simulink model "sampleModel1553"  (R2023a)
settings: Solver=VariableStepAuto  StartTime=0.0  StopTime=10.0  RelTol=1e-3
libraries: hdlsllib x5, simulink x2
settings Model: Creator=user1  LastModifiedBy=user1

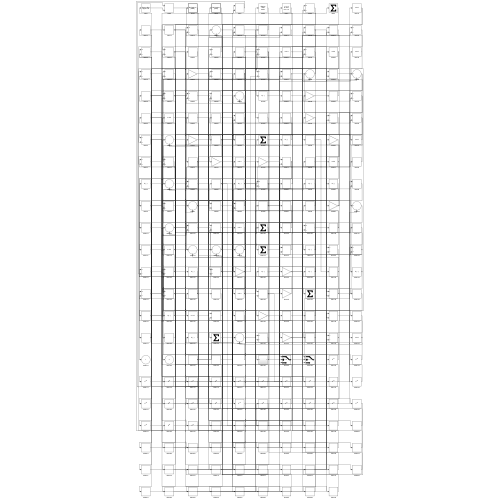
[thumbnail: Simulink's stored preview of the top-level diagram]
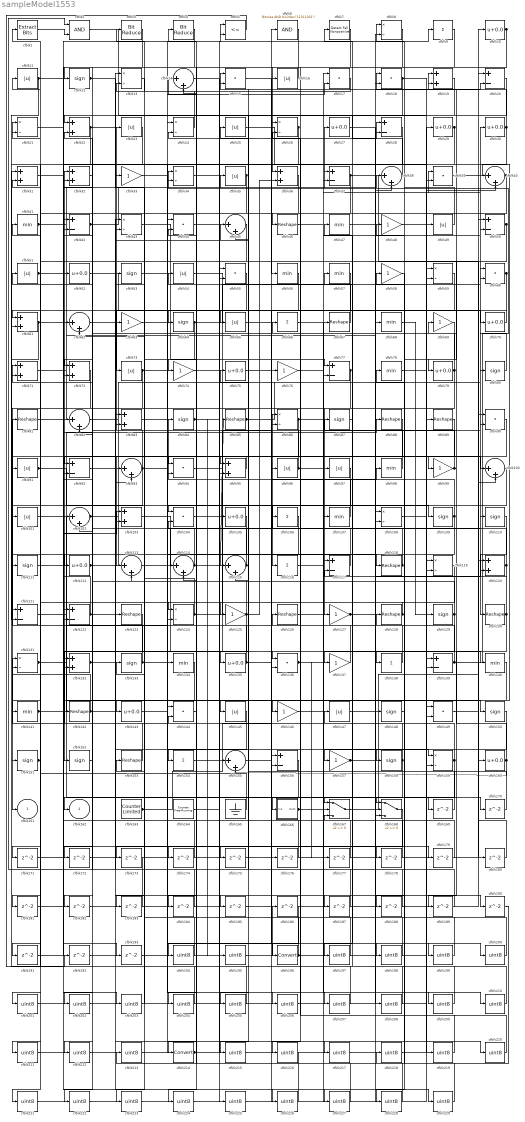
== system sampleModel1553 ==
  cfblk1 : simulink/Logic and Bit Operations/Extract Bits  bitsToExtract=Upper half  numBits=8  bitIdxRange=[0 7]  outScalingMode=Preserve fixed-point scaling
      settings: LibrarySourceBlock=|
      | hdlsllib/Logic and Bit
      | Operations/Extract Bits
  cfblk{10,27,29..30,52,70,75,79,105,112,135,143,160} (13 alike) : Bias  Bias=0.0  SaturateOnIntegerOverflow=off
  cfblk{14,38,40,45,62,82,93,100,102,113..115,155} (13 alike) : Sum  Inputs=|++
  cfblk{11,16,23,25,35,49,51,54,65,73,91,96..97,101,145,147} (16 alike) : Abs  SaturateOnIntegerOverflow=off
  cfblk{19,22,31..32,36,61,71..72,83,95,103,120,132} (13 alike) : Sum
  cfblk{15,17..18,39,44,55,60,90,94,104,136,144,149} (13 alike) : DotProduct  OutDataTypeStr=Inherit: Inherit via internal rule
  cfblk{9,66,106,116,138,154} (6 alike) : Sum  Inputs=+
  cfblk{41,47,56..57,68,78,98,107,134,140..141} (11 alike) : MinMax
  cfblk{8,13,21,24,26,34,43,59,86,108,119,124,131,159} (14 alike) : Product  Inputs=*/  RndMeth=Zero  SaturateOnIntegerOverflow=on
  cfblk{12,53,64,80,84,87,109..111,129,133,148,150..152,158} (16 alike) : Signum
  cfblk{20,28,37,42,50,77,92,117,121..122,139,156} (12 alike) : Sum  Inputs=+-
  cfblk{46,67,81,85,88..89,118,123,126,128,130,142,153} (13 alike) : Reshape
  cfblk{33,48,58,63,69,74,76,99,125,127,137,146,157} (13 alike) : Gain
  cfblk163 : hdlsllib/Sources/Counter Limited  uplimit=7  tsamp=-1
  cfblk164 : hdlsllib/Sources/Counter Free-Running  NumBits=16  tsamp=-1
  cfblk165 : Ground
  cfblk166 : Subsystem
      settings: LibrarySourceBlock=|
      | hdlsllib/Ports &
      | Subsystems/Subsystem
  cfblk167 : Switch  SaturateOnIntegerOverflow=off  InputSameDT=off
  cfblk168 : Switch  SaturateOnIntegerOverflow=off  InputSameDT=off
  cfblk{169..193} (25 alike) : Delay  SampleTime=1
  cfblk{194..195,197..213,215..229} (34 alike) : DataTypeConversion  OutDataTypeStr=uint8  SaturateOnIntegerOverflow=off  RndMeth=Floor
  cfblk196 : DataTypeConversion  SaturateOnIntegerOverflow=off  RndMeth=Floor
  cfblk2 : Logic  AllPortsSameDT=off  OutDataTypeStr=boolean
  cfblk214 : DataTypeConversion  SaturateOnIntegerOverflow=off  RndMeth=Floor
  cfblk3 : hdlsllib/Logic and Bit Operations/Bit Reduce  mode=AND
  cfblk4 : hdlsllib/Logic and Bit Operations/Bit Reduce  mode=AND
  cfblk5 : RelationalOperator  Operator=<=  OutDataTypeStr=boolean  InputSameDT=off
  cfblk6 : simulink/Logic and Bit Operations/Bitwise Operator  logicop=AND  UseBitMask=on  BitMask=bin2dec('11011001')  BitMaskRealWorld=Stored Integer
      settings: LibrarySourceBlock=|
      | hdlsllib/Logic and Bit
      | Operations/Bitwise
      | Operator
  cfblk7 : hdlsllib/Logic and Bit Operations/Detect Fall Nonpositive  vinit=0  OutDataTypeStr=boolean
  cfblk161 : Outport  VectorParamsAs1DForOutWhenUnconnected=off
  cfblk162 : Outport  Port=2  VectorParamsAs1DForOutWhenUnconnected=off
  wires:
  cfblk70/1 -> cfblk61/1
  cfblk84/1 -> cfblk187/1, cfblk195/1
  cfblk77/1 -> cfblk127/1, cfblk124/2
  cfblk139/1 -> cfblk34/1, cfblk103/2
  cfblk73/1 -> cfblk161/1, cfblk199/1
  cfblk54/1 -> cfblk138/1
  cfblk39/1 -> cfblk145/1
  cfblk12/1 -> cfblk217/1, cfblk226/1
  cfblk68/1 -> cfblk129/1
  cfblk26/1 -> cfblk191/1, cfblk205/1, cfblk211/1
  cfblk16/1 -> cfblk12/1
  cfblk122/1 -> cfblk32/1, cfblk123/1
  cfblk98/1 -> cfblk23/1
  cfblk130/1 -> cfblk30/1, cfblk189/1
  cfblk111/1 -> cfblk146/1
  cfblk2/1 -> cfblk119/1
  cfblk22/1 -> cfblk150/1, cfblk93/2, cfblk121/2
  cfblk72/1 -> cfblk151/1
  cfblk103/1 -> cfblk136/1
  cfblk43/1 -> cfblk77/1
  cfblk114/1 -> cfblk85/1, cfblk53/1
  cfblk96/1 -> cfblk75/1, cfblk50/2, cfblk60/2
  cfblk6/1 -> cfblk36/1
  cfblk74/1 -> cfblk9/1
  cfblk158/1 -> cfblk131/1, cfblk184/1
  cfblk143/1 -> cfblk110/1
  cfblk50/1 -> cfblk79/1, cfblk221/1
  cfblk131/1 -> cfblk88/1, cfblk103/1
  cfblk51/1 -> cfblk139/2, cfblk193/1
  cfblk81/1 -> cfblk27/1
  cfblk29/1 -> cfblk46/1, cfblk34/2
  cfblk107/1 -> cfblk84/1
  cfblk15/1 -> cfblk56/1
  cfblk57/1 -> cfblk64/1
  cfblk101/1 -> cfblk167/1
  cfblk75/1 -> cfblk100/1
  cfblk27/1 -> cfblk68/1
  cfblk167/1 -> cfblk50/1
  cfblk7/1 -> cfblk166/1(In1)
  cfblk41/1 -> cfblk13/1, cfblk5/2, cfblk227/1
  cfblk100/1 -> cfblk116/1
  cfblk119/1 -> cfblk141/1
  cfblk69/1 -> cfblk158/1
  cfblk55/1 -> cfblk73/1
  cfblk159/1 -> cfblk62/1, cfblk188/1
  cfblk37/1 -> cfblk160/1, cfblk72/1
  cfblk121/1 -> cfblk143/1
  cfblk123/1 -> cfblk152/1
  cfblk137/1 -> cfblk66/1
  cfblk124/1 -> cfblk6/1, cfblk62/2, cfblk37/1
  cfblk133/1 -> cfblk81/1, cfblk17/2
  cfblk23/1 -> cfblk92/1
  cfblk49/1 -> cfblk18/1
  cfblk19/1 -> cfblk107/1
  cfblk89/1 -> cfblk91/1
  cfblk83/1 -> cfblk38/1
  cfblk164/1 -> cfblk115/1
  cfblk1/1 -> cfblk2/2
  cfblk144/1 -> cfblk4/1
  cfblk56/1 -> cfblk162/1
  cfblk150/1 -> cfblk157/1
  cfblk78/1 -> cfblk140/1
  cfblk128/1 -> cfblk125/1, cfblk78/1
  cfblk97/1 -> cfblk104/1
  cfblk141/1 -> cfblk24/1, cfblk35/1
  cfblk46/1 -> cfblk28/1
  cfblk99/1 -> cfblk69/1, cfblk45/2
  cfblk85/1 -> cfblk49/1, cfblk200/1
  cfblk165/1 -> cfblk41/1
  cfblk35/1 -> cfblk154/1, cfblk224/1
  cfblk38/1 -> cfblk7/1
  cfblk60/1 -> cfblk112/1, cfblk86/2
  cfblk18/1 -> cfblk89/1, cfblk215/1
  cfblk135/1 -> cfblk98/1, cfblk21/1
  cfblk11/1 -> cfblk61/2, cfblk39/2
  cfblk138/1 -> cfblk128/1
  cfblk8/1 -> cfblk124/1
  cfblk166/1(Out1) -> cfblk90/2, cfblk26/2
  cfblk120/1 -> cfblk86/1, cfblk117/2
  cfblk118/1 -> cfblk51/1, cfblk87/1
  cfblk61/1 -> cfblk111/1, cfblk99/1, cfblk71/2, cfblk179/1
  cfblk17/1 -> cfblk13/2
  cfblk33/1 -> cfblk196/1
  cfblk82/1 -> cfblk10/1
  cfblk67/1 -> cfblk54/1
  cfblk148/1 -> cfblk8/1
  cfblk25/1 -> cfblk38/2
  cfblk153/1 -> cfblk11/1
  cfblk112/1 -> cfblk67/1, cfblk92/2
  cfblk109/1 -> cfblk115/2, cfblk48/1, cfblk15/2
  cfblk151/1 -> cfblk131/2, cfblk121/1
  cfblk132/1 -> cfblk159/1, cfblk168/3
  cfblk142/1 -> cfblk168/1, cfblk21/2
  cfblk152/1 -> cfblk82/1
  cfblk110/1 -> cfblk130/1
  cfblk116/1 -> cfblk80/1
  cfblk9/1 -> cfblk94/1
  cfblk126/1 -> cfblk149/2
  cfblk93/1 -> cfblk101/1, cfblk5/1, cfblk71/1
  cfblk129/1 -> cfblk137/1, cfblk113/2
  cfblk40/1 -> cfblk135/1, cfblk65/1
  cfblk113/1 -> cfblk100/2
  cfblk80/1 -> cfblk60/1
  cfblk64/1 -> cfblk37/2, cfblk207/1, cfblk223/1
  cfblk160/1 -> cfblk19/1, cfblk155/2
  cfblk20/1 -> cfblk102/2
  cfblk136/1 -> cfblk40/1, cfblk177/1
  cfblk86/1 -> cfblk170/1, cfblk171/1
  cfblk3/1 -> cfblk22/1
  cfblk42/1 -> cfblk16/1, cfblk70/1
  cfblk48/1 -> cfblk40/2
  cfblk53/1 -> cfblk118/1
  cfblk115/1 -> cfblk32/2, cfblk25/1
  cfblk28/1 -> cfblk94/2
  cfblk163/1 -> cfblk96/1, cfblk28/2
  cfblk45/1 -> cfblk74/1
  cfblk94/1 -> cfblk148/1
  cfblk79/1 -> cfblk42/1, cfblk132/2
  cfblk30/1 -> cfblk132/1, cfblk15/1
  cfblk106/1 -> cfblk214/1
  cfblk147/1 -> cfblk39/1
  cfblk157/1 -> cfblk20/2, cfblk19/2
  cfblk88/1 -> cfblk113/1
  cfblk10/1 -> cfblk142/1, cfblk114/2
  cfblk87/1 -> cfblk57/1
  cfblk52/1 -> cfblk139/1
  cfblk102/1 -> cfblk43/1, cfblk109/1
  cfblk24/1 -> cfblk3/1
  cfblk95/1 -> cfblk93/1
  cfblk71/1 -> cfblk8/2
  cfblk91/1 -> cfblk155/1, cfblk95/1
  cfblk127/1 -> cfblk120/2, cfblk169/1
  cfblk117/1 -> cfblk83/2
  cfblk155/1 -> cfblk136/2
  cfblk4/1 -> cfblk122/2
  cfblk125/1 -> cfblk52/1, cfblk36/2, cfblk182/1
  cfblk169/1 -> cfblk43/2
  cfblk170/1 -> cfblk24/2
  cfblk171/1 -> cfblk77/2
  cfblk32/1 -> cfblk172/1
  cfblk172/1 -> cfblk90/1
  cfblk168/1 -> cfblk173/1
  cfblk173/1 -> cfblk2/1
  cfblk21/1 -> cfblk174/1
  cfblk174/1 -> cfblk122/1
  cfblk92/1 -> cfblk175/1
  cfblk175/1 -> cfblk18/2
  cfblk65/1 -> cfblk176/1
  cfblk176/1 -> cfblk102/1
  cfblk177/1 -> cfblk22/2
  cfblk146/1 -> cfblk178/1
  cfblk178/1 -> cfblk167/2
  cfblk179/1 -> cfblk167/3
  cfblk149/1 -> cfblk180/1
  cfblk180/1 -> cfblk20/1
  cfblk36/1 -> cfblk181/1
  cfblk181/1 -> cfblk114/1
  cfblk182/1 -> cfblk95/2
  cfblk13/1 -> cfblk183/1
  cfblk183/1 -> cfblk83/1
  cfblk184/1 -> cfblk82/2
  cfblk62/1 -> cfblk185/1
  cfblk185/1 -> cfblk120/1
  cfblk187/1 -> cfblk1/1
  cfblk188/1 -> cfblk72/2
  cfblk189/1 -> cfblk45/1
  cfblk66/1 -> cfblk190/1
  cfblk191/1 -> cfblk42/2
  cfblk5/1 -> cfblk192/1
  cfblk192/1 -> cfblk117/1
  cfblk193/1 -> cfblk119/2
  cfblk186/1 -> cfblk194/1
  cfblk194/1 -> cfblk144/1
  cfblk195/1 -> cfblk186/1
  cfblk196/1 -> cfblk168/2, cfblk144/2
  cfblk90/1 -> cfblk197/1
  cfblk197/1 -> cfblk33/1
  cfblk44/1 -> cfblk198/1
  cfblk198/1 -> cfblk26/1
  cfblk199/1 -> cfblk44/1
  cfblk200/1 -> cfblk44/2
  cfblk105/1 -> cfblk201/1
  cfblk201/1 -> cfblk17/1
  cfblk140/1 -> cfblk202/1
  cfblk202/1 -> cfblk105/1
  cfblk31/1 -> cfblk203/1
  cfblk203/1 -> cfblk133/1
  cfblk145/1 -> cfblk204/1
  cfblk204/1 -> cfblk31/1
  cfblk205/1 -> cfblk31/2
  cfblk63/1 -> cfblk206/1
  cfblk206/1 -> cfblk29/1
  cfblk207/1 -> cfblk63/1
  cfblk47/1 -> cfblk208/1
  cfblk208/1 -> cfblk147/1
  cfblk154/1 -> cfblk209/1
  cfblk209/1 -> cfblk47/1
  cfblk76/1 -> cfblk210/1
  cfblk210/1 -> cfblk153/1
  cfblk211/1 -> cfblk76/1
  cfblk134/1 -> cfblk212/1
  cfblk212/1 -> cfblk55/1
  cfblk213/1 -> cfblk134/1
  cfblk214/1 -> cfblk55/2, cfblk159/2
  cfblk215/1 -> cfblk106/1
  cfblk59/1 -> cfblk216/1
  cfblk216/1 -> cfblk213/1
  cfblk217/1 -> cfblk59/1
  cfblk190/1 -> cfblk218/1
  cfblk218/1 -> cfblk59/2
  cfblk108/1 -> cfblk219/1
  cfblk219/1 -> cfblk126/1
  cfblk104/1 -> cfblk220/1
  cfblk220/1 -> cfblk108/1
  cfblk221/1 -> cfblk108/2
  cfblk156/1 -> cfblk222/1
  cfblk222/1 -> cfblk149/1
  cfblk223/1 -> cfblk156/1
  cfblk224/1 -> cfblk156/2
  cfblk14/1 -> cfblk225/1
  cfblk225/1 -> cfblk97/1
  cfblk226/1 -> cfblk14/1
  cfblk227/1 -> cfblk14/2
  cfblk58/1 -> cfblk228/1
  cfblk228/1 -> cfblk104/2
  cfblk34/1 -> cfblk229/1
  cfblk229/1 -> cfblk58/1

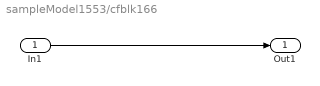
== system sampleModel1553/cfblk166 ==
  In1 : Inport
  Out1 : Outport
  wires:
  In1/1 -> Out1/1
